simulink model "Iastar"  (R2016a)
settings: Solver=VariableStepAuto  StartTime=0.0  StopTime=10.0  RelTol=1e-3
undefined symbols (not defined in the file): Tg
settings Model: Creator=hi  LastModifiedBy=hi

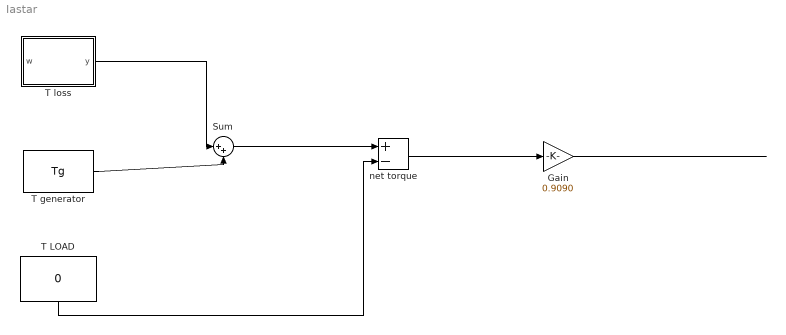
== system Iastar ==
  Gain : Gain  Gain=0.9090
  Sum : Sum  Inputs=|++
  T LOAD : Constant  Value=0
  T generator : Constant  Value=Tg
  T loss : MATLAB Function  TreatAsAtomicUnit=on
  net torque : Sum  Inputs=+-
  wires:
  T LOAD/1 -> net torque/2
  T loss/1(y) -> Sum/1
  T generator/1 -> Sum/2
  Sum/1 -> net torque/1
  net torque/1 -> Gain/1
  Gain/1 -> ?

== matlab function Iastar/T loss ==
  data: w input; y output
function y = fcn(w)
%#codegen

y = 0.0023w+0.418;
